simulink library "INT_EGRVlv_DDSens"  (R2016b)
settings: Solver=VariableStepAuto  StartTime=0.0  StopTime=10.0  RelTol=1e-3
settings Model: Creator=zhulinfeng  LastModifiedBy=zhulinfeng

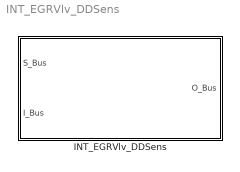
== system INT_EGRVlv_DDSens ==
  INT_EGRVlv_DDSens : Subsystem

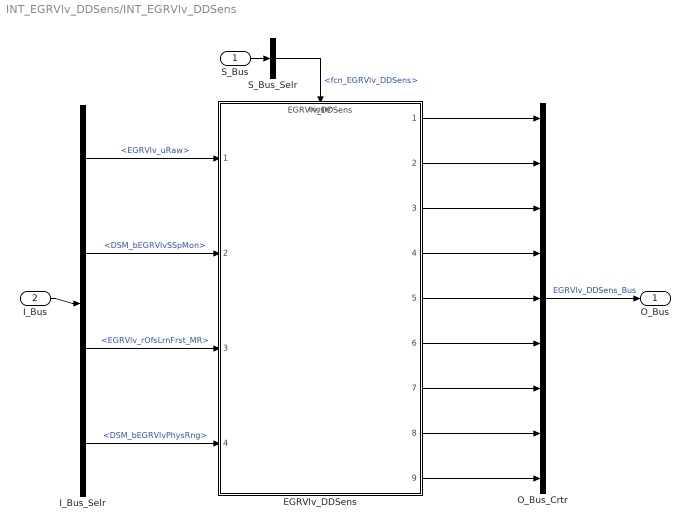
== system INT_EGRVlv_DDSens/INT_EGRVlv_DDSens ==
  S_Bus : Inport
  I_Bus : Inport  Port=2
  EGRVlv_DDSens : ModelReference  ModelNameDialog=EGRVlv_DDSens  SimulationMode=Normal  ModelReferenceVersion=1.13  TriggerPortName=function  TriggerPortTriggerType=function-call  TriggerPortStatesWhenEnabling=held
  I_Bus_Selr : BusSelector  OutputSignals=EGRVlv_uRaw,DSM_bEGRVlvSSpMon,EGRVlv_rOfsLrnFrst_MR,DSM_bEGRVlvPhysRng
  O_Bus_Crtr : BusCreator  Inputs=9
  S_Bus_Selr : BusSelector  OutputSignals=fcn_EGRVlv_DDSens
  O_Bus : Outport
  wires:
  S_Bus_Selr/1 -> EGRVlv_DDSens/Trigger  "<fcn_EGRVlv_DDSens>"
  S_Bus/1 -> S_Bus_Selr/1
  I_Bus/1 -> I_Bus_Selr/1
  I_Bus_Selr/1 -> EGRVlv_DDSens/1  "<EGRVlv_uRaw>"
  I_Bus_Selr/2 -> EGRVlv_DDSens/2  "<DSM_bEGRVlvSSpMon>"
  I_Bus_Selr/3 -> EGRVlv_DDSens/3  "<EGRVlv_rOfsLrnFrst_MR>"
  I_Bus_Selr/4 -> EGRVlv_DDSens/4  "<DSM_bEGRVlvPhysRng>"
  O_Bus_Crtr/1 -> O_Bus/1  "EGRVlv_DDSens_Bus"
  EGRVlv_DDSens/1 -> O_Bus_Crtr/1
  EGRVlv_DDSens/2 -> O_Bus_Crtr/2
  EGRVlv_DDSens/3 -> O_Bus_Crtr/3
  EGRVlv_DDSens/4 -> O_Bus_Crtr/4
  EGRVlv_DDSens/5 -> O_Bus_Crtr/5
  EGRVlv_DDSens/6 -> O_Bus_Crtr/6
  EGRVlv_DDSens/7 -> O_Bus_Crtr/7
  EGRVlv_DDSens/8 -> O_Bus_Crtr/8
  EGRVlv_DDSens/9 -> O_Bus_Crtr/9
